simulink model "q_qube2_bal_lqr_swing_up_funzionanteeeeeee"  (R2020b)
settings: Solver=ode1  StartTime=0.0  StopTime=10  FixedStep=0.002  RelTol=1e-3  EnableMultiTasking=on
undefined symbols (not defined in the file): HIL, K, qc_get_step_size
libraries: simulink_extras x3, simulink x3, quarc_library x3
settings Model: SimulationMode=external  ExtModeTrigDuration=10000  Creator=MLevis  LastModifiedBy=marco
settings SolverCC: PositivePriorityOrder=on
settings DataIOCC: LimitDataPoints=on  SaveFormat=Array  SignalLoggingSaveFormat=ModelDataLogs  ReturnWorkspaceOutputs=off
settings OptimizationCC: BooleanDataType=off  OptimizeBlockIOStorage=off  BufferReuse=off  GlobalBufferReuse=off  ExpressionFolding=off  ExpressionDepthLimit=2147483647  LocalBlockOutputs=off  InitFltsAndDblsToZero=on  LifeSpan=inf  OptimizeDataStoreBuffers=off  BusAssignmentInplaceUpdate=off
settings DebuggingCC: SaveWithParameterizedLinksMsg=none  UnderspecifiedInitializationDetection=Classic  MergeDetectMultiDrivingBlocksExec=none  SignalResolutionControl=TryResolveAllWithWarning  MultiTaskDSMMsg=warning  MultiTaskCondExecSysMsg=none  FcnCallInpInsideContextMsg=warning  StateNameClashWarn=warning  SFUnexpectedBacktrackingDiag=warning  SFNoUnconditionalDefaultTransitionDiag=warning  SFExecutionAtInitializationDiag=none  ArithmeticOperatorsInVariantConditions=warning
settings HardwareCC: ProdBitPerPointer=32  ProdBitPerSizeT=32  ProdBitPerPtrDiffT=32  ProdLargestAtomicFloat=None  ProdIntDivRoundTo=Undefined  ProdEndianess=Unspecified  ProdWordSize=32  ProdHWDeviceType=32-bit Generic  TargetHWDeviceType=32-bit Generic
settings ModelReferenceCC: PropagateSignalLabelsOutOfModel=off
settings SFSimCC: SimUseLocalCustomCode=off  SimParseCustomCode=off  CustomCodeUndefinedFunction=UseInterfaceOnly
settings RTWCC: Description=QUARC Win64 Target  SystemTargetFile=quarc_win64.tlc  TemplateMakefile=quarc_default_tmf  RTWUseLocalCustomCode=off
settings CodeAppCC: StateflowObjectComments=on
settings STFCustomTargetCC: CPPClassGenCompliant=off
settings GRTTargetCC: TargetLangStandard=C89/C90 (ANSI)  ParMdlRefBuildCompliant=off  CompOptLevelCompliant=off  CombineOutputUpdateFcns=off  MatFileLogging=off  CPPClassGenCompliant=off  GRTInterface=on  UseToolchainInfoCompliant=off  ExtMode=on  ExtModeMexFile=quarc_comm
settings ConfigComp: CovMetricSettings=dw  CovSaveCumulativeToWorkspaceVar=on  CovSaveSingleToWorkspaceVar=on  CovExternalEMLEnable=off  CovSFcnEnable=off

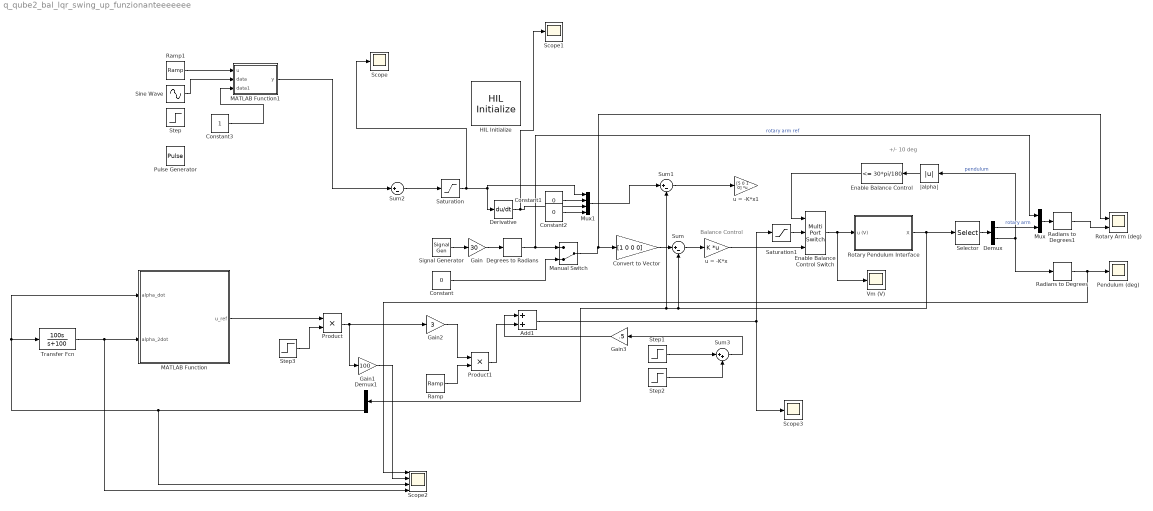
== system q_qube2_bal_lqr_swing_up_funzionanteeeeeee ==
  note: +/- 10 deg
  note: Balance Control
  Add1 : Sum
  Constant : Constant  Value=0
  Constant1 : Constant  Value=0
  Constant2 : Constant  Value=0
  Constant3 : Constant
  Convert to Vector : Gain  Gain=[1 0 0 0]
  Degrees to Radians : simulink_extras/Transformations/Degrees to Radians
  Demux : Demux  Outputs=2
  Demux1 : Demux
  Derivative : Derivative
  Enable Balance Control : simulink/Logic and Bit Operations/Compare To Constant  relop=<=  const=30*pi/180  OutDataTypeStr=uint8  ZeroCross=off
  Enable Balance Control Switch : MultiPortSwitch  DataPortOrder=Zero-based contiguous  Inputs=2  zeroidx=on
  Gain : Gain  Gain=30
  Gain1 : Gain  Gain=100
  Gain2 : Gain  Gain=3
  Gain3 : Gain  Gain=.5
  HIL Initialize : quarc_library/Data Acquisition/Generic/Configuration/HIL Initialize  object_name=HIL-1  board_type=qube_servo2_usb  board_number=0  board_options=""  exclusive=off  active=off  hardware_clocks=[0]  clock_modes=[]  initial_clock_frequencies=[]  set_clock_params_at_start=off  set_clock_params_at_switch_in=off  set_clock_frequencies_at_start=off  set_clock_frequencies_at_switch_in=off  analog_input_channels=[0]  analog_input_configurations=[]  analog_input_maximums=3  analog_input_minimums=-3  set_analog_input_params_at_start=off  set_analog_input_params_at_switch_in=off  analog_output_channels=[0]  analog_output_maximums=15  analog_output_minimums=-15  initial_analog_outputs=[0]  final_analog_outputs=[0]  watchdog_analog_outputs=0  set_analog_output_params_at_start=off  set_analog_output_params_at_switch_in=off  set_analog_outputs_at_start=on  set_analog_outputs_at_switch_in=off  set_analog_outputs_at_terminate=on  set_analog_outputs_at_switch_out=off  set_analog_outputs_on_watchdog=on  digital_input_channels=[]  digital_output_channels=[0]  digital_output_configuration=[]  initial_digital_outputs=[1]  final_digital_outputs=[0]  watchdog_digital_outputs=[0]  set_digital_output_params_at_start=off  set_digital_output_params_at_switch_in=off  set_digital_outputs_at_start=on  set_digital_outputs_at_switch_in=off  set_digital_outputs_at_terminate=on  set_digital_outputs_at_switch_out=off  set_digital_outputs_on_watchdog=on  encoder_channels=[0:1]  quadrature=[4]  encoder_filter_frequency=[]  initial_encoder_counts=[0]  set_encoder_params_at_start=off  set_encoder_params_at_switch_in=off  set_encoder_counts_at_start=on  set_encoder_counts_at_switch_in=off  pwm_channels=[]  pwm_modes=[]  pwm_frequency=[]  pwm_configuration=[]  pwm_alignment=[]  pwm_polarity=[]  pwm_leading_deadband=[]  pwm_trailing_deadband=[]  initial_pwm_outputs=[]  final_pwm_outputs=[]  watchdog_pwm_outputs=[]  set_pwm_params_at_start=off  set_pwm_params_at_switch_in=off  set_pwm_outputs_at_start=off  set_pwm_outputs_at_switch_in=off  set_pwm_outputs_at_terminate=off  set_pwm_outputs_at_switch_out=off  set_pwm_outputs_on_watchdog=off  other_output_channels=[11000:11002]  initial_other_outputs=[0 1 0]  final_other_outputs=[1 0 0]  watchdog_other_outputs=[0 0 1]  set_other_outputs_at_start=on  set_other_outputs_at_switch_in=off  set_other_outputs_at_terminate=on  set_other_outputs_at_switch_out=off  set_other_outputs_on_watchdog=on
  MATLAB Function : MATLAB Function  TreatAsAtomicUnit=on
  MATLAB Function1 : MATLAB Function  TreatAsAtomicUnit=on
  Manual Switch : ManualSwitch  CurrentSetting=0
  Mux : Mux  Inputs=2
  Mux1 : Mux
  Pendulum (deg) : Scope
  Product : Product
  Product1 : Product
  Pulse Generator : DiscretePulseGenerator  PulseType=Time based  Period=.72  PulseWidth=90
  Radians to Degrees : simulink_extras/Transformations/Radians to Degrees
  Radians to Degrees1 : simulink_extras/Transformations/Radians to Degrees
  Ramp : simulink/Sources/Ramp  slope=0.8  start=2  InitialOutput=0
  Ramp1 : simulink/Sources/Ramp  slope=.5  start=1  InitialOutput=0
  Rotary Arm (deg) : Scope  NumInputPorts=2
  Rotary Pendulum Interface : Subsystem
  Saturation : Saturate  UpperLimit=.7  LowerLimit=-.7
  Saturation1 : Saturate  UpperLimit=15  LowerLimit=-15
  Scope : Scope
  Scope1 : Scope
  Scope2 : Scope  NumInputPorts=4
  Scope3 : Scope
  Selector : Selector  InputPortWidth=4  IndexOptions=Index vector (dialog)  Indices=[1 2]  OutputSizes=1
  Signal Generator : SignalGenerator  WaveForm=square  Frequency=0.125
  Sine Wave : Sin  Frequency=8.72  SampleTime=0
  Step : Step  Time=3.922  Before=1  After=0  SampleTime=0
  Step1 : Step  Time=2  After=5  SampleTime=0
  Step2 : Step  Time=2.1  After=-5  SampleTime=0
  Step3 : Step  SampleTime=0
  Sum : Sum  Inputs=|+-
  Sum1 : Sum  Inputs=|+-
  Sum2 : Sum  Inputs=|+-
  Sum3 : Sum  Inputs=|++
  Transfer Fcn : TransferFcn  Numerator=[100 0]  Denominator=[1 100]
  Vm (V) : Scope
  u = -K*x : Gain  Gain=K  Multiplication=Matrix(K*u)
  u = -K*x1 : Gain  Gain=[5 0 1 0]  Multiplication=Matrix(K*u)
  |alpha| : Abs
  wires:
  |alpha|/1 -> Enable Balance Control/1
  Enable Balance Control/1 -> Enable Balance Control Switch/1
  Sum/1 -> u = -K*x/1
  u = -K*x/1 -> Enable Balance Control Switch/3
  Convert to Vector/1 -> Sum/1
  Radians to Degrees/1 -> Scope2/1, Pendulum (deg)/1
  Radians to Degrees1/1 -> Rotary Arm (deg)/2
  Enable Balance Control Switch/1 -> Vm (V)/1, Rotary Pendulum Interface/1(u (V))
  Signal Generator/1 -> Gain/1
  Gain/1 -> Degrees to Radians/1
  Mux/1 -> Radians to Degrees1/1
  Rotary Pendulum Interface/1(X) -> Selector/1, Demux1/1, Sum1/2, Sum/2
  Selector/1 -> Demux/1
  Demux/1 -> Mux/2  "rotary arm"
  Demux/2 -> Radians to Degrees/1, |alpha|/1  "pendulum"
  Degrees to Radians/1 -> Mux/1, Manual Switch/1  "rotary arm ref"
  Manual Switch/1 -> Rotary Arm (deg)/1, Convert to Vector/1
  Constant/1 -> Manual Switch/2
  Sum1/1 -> u = -K*x1/1
  Mux1/1 -> Sum1/1
  Constant1/1 -> Mux1/2
  Constant2/1 -> Mux1/4
  Saturation/1 -> Scope/1, Mux1/1, Derivative/1
  Derivative/1 -> Scope1/1, Mux1/3
  Sine Wave/1 -> MATLAB Function1/2(data)
  MATLAB Function1/1(y) -> Sum2/1
  Ramp1/1 -> MATLAB Function1/1(u)
  Sum2/1 -> Saturation/1
  Constant3/1 -> MATLAB Function1/3(data1)
  Step2/1 -> Sum3/2
  Step1/1 -> Sum3/1
  Sum3/1 -> Gain3/1
  Add1/1 -> Scope3/1, Saturation1/1
  Demux1/4 -> Scope2/3, MATLAB Function/1(alpha_dot), Transfer Fcn/1
  Transfer Fcn/1 -> Scope2/4, MATLAB Function/2(alpha_2dot)
  MATLAB Function/1(u_ref) -> Product/1
  Step3/1 -> Product/2
  Gain1/1 -> Scope2/2
  Product/1 -> Gain2/1, Gain1/1
  Gain3/1 -> Add1/1
  Saturation1/1 -> Enable Balance Control Switch/2
  Gain2/1 -> Product1/1
  Ramp/1 -> Product1/2
  Product1/1 -> Add1/2

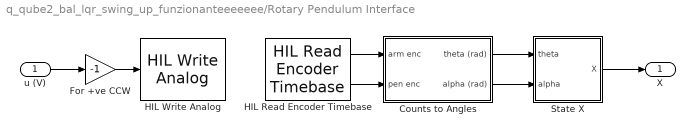
== system q_qube2_bal_lqr_swing_up_funzionanteeeeeee/Rotary Pendulum Interface ==
  u (V) : Inport
  Counts to Angles : Subsystem
  For +ve CCW : Gain  Gain=-1
  HIL Read Encoder Timebase : quarc_library/Data Acquisition/Generic/Timebases/HIL Read Encoder Timebase  object_name=HIL-1  clock=0  channels=[0:1]  active=on  vector_output=off  data_type_mode=Inherit via back propagation  data_type=double  overflow_mode=Error on overflow  samples_in_buffer=max(ceil(1/qc_get_step_size), 1)
  HIL Write Analog : quarc_library/Data Acquisition/Generic/Immediate I//O/HIL Write Analog  object_name=HIL-1  channels=0  sample_time=-1  active=off  vector_input=off
  State X : Subsystem
  X : Outport  VectorParamsAs1DForOutWhenUnconnected=off
  wires:
  u (V)/1 -> For +ve CCW/1
  HIL Read Encoder Timebase/2 -> Counts to Angles/2(pen enc)
  For +ve CCW/1 -> HIL Write Analog/1
  HIL Read Encoder Timebase/1 -> Counts to Angles/1(arm enc)
  Counts to Angles/2(alpha (rad)) -> State X/2(alpha)
  Counts to Angles/1(theta (rad)) -> State X/1(theta)
  State X/1(X) -> X/1

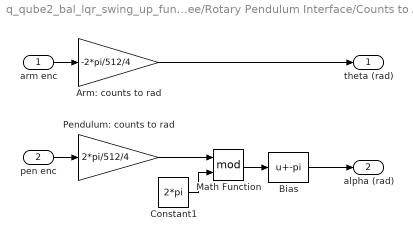
== system q_qube2_bal_lqr_swing_up_funzionanteeeeeee/Rotary Pendulum Interface/Counts to Angles ==
  arm enc : Inport
  pen enc : Inport  Port=2
  Arm: counts to rad : Gain  Gain=-2*pi/512/4
  Bias : Bias  Bias=-pi
  Constant1 : Constant  Value=2*pi
  Math Function : Math  Operator=mod  SignedPower=on  SaturateOnIntegerOverflow=on
  Pendulum: counts to rad : Gain  Gain=2*pi/512/4
  theta (rad) : Outport  VectorParamsAs1DForOutWhenUnconnected=off
  alpha (rad) : Outport  Port=2  VectorParamsAs1DForOutWhenUnconnected=off
  wires:
  pen enc/1 -> Pendulum: counts to rad/1
  arm enc/1 -> Arm: counts to rad/1
  Math Function/1 -> Bias/1
  Constant1/1 -> Math Function/2
  Pendulum: counts to rad/1 -> Math Function/1
  Arm: counts to rad/1 -> theta (rad)/1
  Bias/1 -> alpha (rad)/1

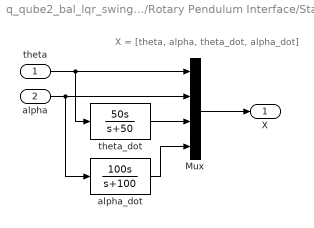
== system q_qube2_bal_lqr_swing_up_funzionanteeeeeee/Rotary Pendulum Interface/State X ==
  note: X = [theta, alpha, theta_dot, alpha_dot]
  theta : Inport
  alpha : Inport  Port=2
  Mux : Mux
  alpha_dot : TransferFcn  Numerator=[100 0]  Denominator=[1 100]
  theta_dot : TransferFcn  Numerator=[50 0]  Denominator=[1 50]
  X : Outport  VectorParamsAs1DForOutWhenUnconnected=off
  wires:
  theta_dot/1 -> Mux/3
  alpha_dot/1 -> Mux/4
  alpha/1 -> Mux/2, alpha_dot/1
  Mux/1 -> X/1
  theta/1 -> Mux/1, theta_dot/1

== matlab function q_qube2_bal_lqr_swing_up_funzionanteeeeeee/MATLAB Function ==
  settings: updateMethod=DISCRETE  sampleTime=0.002
  data: alpha_dot input; u_ref output; alpha_2dot input
%function [u_ref, flag_o, tick_o, started_o]  = fcn(alpha_dot,alpha_2dot)
function u_ref   = fcn(alpha_dot,alpha_2dot)
%% allocazione
%farei una rampa che aumenta sotto certe condizioni e diminuire per altre
persistent  alpha_dot_k_1;
persistent  alpha_2dot_k_1;
persistent tick started;
persistent flag;

if isempty(flag)
    flag = 0;
end

if isempty(tick)
    tick = 0;
end

if isempty(started)
    started = 0;
end 

if isempty(alpha_dot_k_1)
 alpha_dot_k_1   = 0;
end

if isempty(alpha_2dot_k_1)
    alpha_2dot_k_1   = 0;
end


%% inizio codice

y=0;

if flag == 10 %resetto se no aumenta all'infinito --> verificare se è corretto
    flag=0;
end

%if (not(sign(alpha_2dot) == sign(alpha_2dot_k_1)) || alpha_2dot == 0) &&
%(abs(alpha_dot_k_1)>= abs(alpha_dot)) && (not(alpha==180))


if (not(sign(alpha_2dot) == sign(alpha_2dot_k_1)) || alpha_2dot == 0) && (abs(alpha_dot_k_1)>= abs(alpha_dot)) 
    % problema...nel punto a max velocità (più in basso) per rumore potrebbe verificarsi la condizione (se metto alpha diverso da 180 (lo zero è dall'alto) avrei bisogno di un gradino iniziale se no non parte nulla)
     started = 1;
end

if (started == 1)
    if tick < (2e-3*50) 

        tick=tick+2e-3;
        y=1;
        
    else
        flag = flag + 1; %ogni volta che aumenta significa che ho fatto tot ms alti
        tick = 0;
        started = 0;
    end 
else
    y=0;
end 


if y ==1 
    if mod(flag, 2) == 0 
        y=-1;
    else
        y=1;
    end
end

alpha_dot_k_1 = alpha_dot; 
alpha_2dot_k_1 = alpha_2dot; 

u_ref=y;
%flag_o = flag;
%tick_o = tick;
%started_o = started;
end

== matlab function q_qube2_bal_lqr_swing_up_funzionanteeeeeee/MATLAB Function1 ==
  data: u input; y output; data input; data1 input
function y = fcn(u, data, data1)

y = u*data*data1;
